simulink model "vrguiJP_R2012b_wersja2"  (R2019b)
settings: Solver=FixedStepDiscrete  StartTime=0.0  StopTime=inf  RelTol=1e-3  EnableMultiTasking=on
undefined symbols (not defined in the file): gray, pause, strel
libraries: visionanalysis x3, visiontextngfix x2, visionstatistics x1, visionmorphops x1, dspvision x1, visiongeotforms x1
settings Model: Creator=Tomek  LastModifiedBy=fw2ty
settings DataIOCC: LimitDataPoints=on  SaveFormat=Array  SignalLoggingSaveFormat=ModelDataLogs  ReturnWorkspaceOutputs=off
settings OptimizationCC: ExpressionDepthLimit=2147483647  InitFltsAndDblsToZero=on  LifeSpan=inf
settings DebuggingCC: SaveWithParameterizedLinksMsg=none  UnderspecifiedInitializationDetection=Classic  MergeDetectMultiDrivingBlocksExec=none  SignalResolutionControl=TryResolveAllWithWarning  MultiTaskDSMMsg=warning  MultiTaskCondExecSysMsg=none  FcnCallInpInsideContextMsg=warning  StateNameClashWarn=warning  SFUnexpectedBacktrackingDiag=warning  SFNoUnconditionalDefaultTransitionDiag=warning  SFExecutionAtInitializationDiag=none  ArithmeticOperatorsInVariantConditions=warning
settings HardwareCC: ProdBitPerPointer=32  ProdBitPerSizeT=32  ProdBitPerPtrDiffT=32  ProdLargestAtomicFloat=None  ProdIntDivRoundTo=Undefined  ProdEndianess=Unspecified  ProdWordSize=32  ProdHWDeviceType=32-bit Generic  TargetHWDeviceType=32-bit Generic  TargetUnknown=on  ProdEqTarget=off
settings ModelReferenceCC: PropagateSignalLabelsOutOfModel=off
settings SFSimCC: SimUseLocalCustomCode=off  SimParseCustomCode=off  CustomCodeUndefinedFunction=UseInterfaceOnly
settings RTWCC: RTWUseLocalCustomCode=off
settings CodeAppCC: StateflowObjectComments=on
settings GRTTargetCC: TargetFcnLib=ansi_tfl_tmw.mat  TargetLangStandard=C89/C90 (ANSI)  GeneratePreprocessorConditionals=Disable all  CombineOutputUpdateFcns=off  GRTInterface=on
settings ConfigComp: CovMetricSettings=dw  CovHtmlReporting=on  CovSaveCumulativeToWorkspaceVar=on  CovSaveSingleToWorkspaceVar=on  CovExternalEMLEnable=off

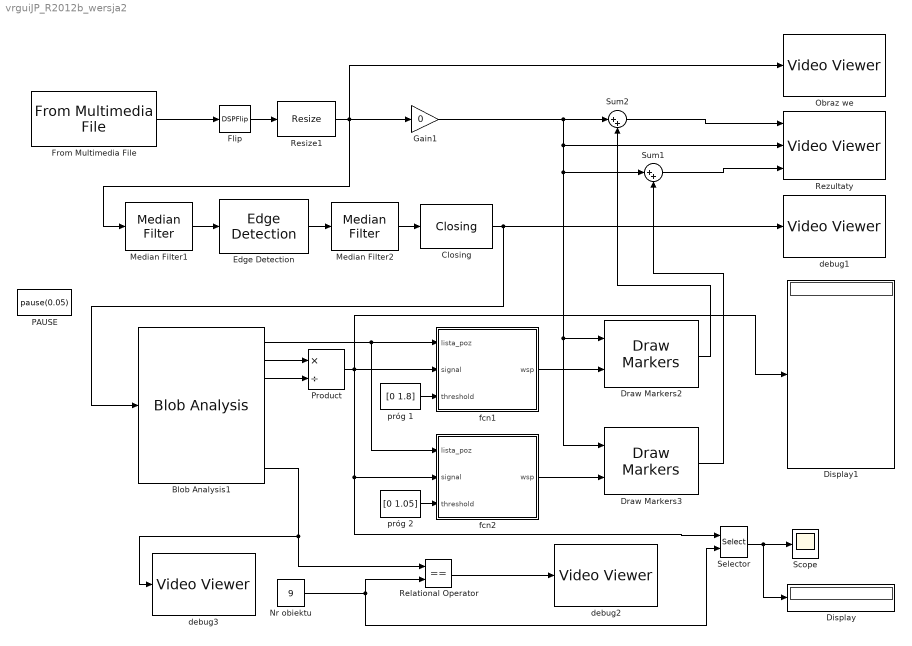
== system vrguiJP_R2012b_wersja2 ==
  Blob Analysis1 : visionstatistics/Blob Analysis  Tag=vipblks_row_conv  area=off  centroid=on  bBox=off  majorAxis=on  minorAxis=on  angle=off  eccentricity=on  equivDiameterSq=on  extent=on  perimeter=on  outDT=double  conn=8  isLabel=on  maxBlobs=10  warnIfNumBlobsExceeded=on  isCount=off  useMinArea=on  minArea=45  useMaxArea=off  maxArea=intmax('uint32')  excludeBorderBlob=on  isOutVarDim=off  isFill=on  fillValues=-1  roundingMode=Floor  overflowMode=off  prodOutputMode=Binary point scaling  prodOutputWordLength=32  prodOutputFracLength=16  prodOutputSlope=2^-16  accumMode=Binary point scaling  accumWordLength=32  accumFracLength=0  accumSlope=2^0  outputMode=Binary point scaling  outputWordLength=32  outputFracLength=16  outputSlope=2^-16  memorySlope=2^-16  firstCoeffMode=Binary point scaling  firstCoeffWordLength=16  firstCoeffFracLength=14  firstCoeffSlope=2^-14  secondCoeffMode=Binary point scaling  secondCoeffWordLength=32  secondCoeffFracLength=16  secondCoeffSlope=2^-16
      settings: SourceProductName=Computer Vision Toolbox
  Closing : visionmorphops/Closing  nhoodsrc=Specify via dialog  strel=strel('line',5,45)
      settings: SourceProductName=Computer Vision Toolbox  SourceProductBaseCode=VP
  Display : Display
  Display1 : Display
  Draw Markers2 : visiontextngfix/Draw Markers  shape=Circle  size=10  fill=on  fillClrSource=Specify via dialog  display=White  intensity=200  color=[200 255 100]  opacity=0.5  viewport=Entire image  antialiasing=off  inType=Obsolete  imagePorts=One multidimensional signal  roundingMode=Floor  overflowMode=off  memoryMode=Specify word length  memoryWordLength=16  memoryFracLength=14  memorySlope=2^-14  prodOutputMode=Binary point scaling  prodOutputWordLength=32  prodOutputFracLength=14  prodOutputSlope=2^-14  accumSlope=2^-14
      settings: SourceProductName=Computer Vision Toolbox  SourceProductBaseCode=VP
  Draw Markers3 : visiontextngfix/Draw Markers  shape=Circle  size=10  fill=on  fillClrSource=Specify via dialog  display=White  intensity=200  color=[200 255 100]  opacity=0.5  viewport=Entire image  antialiasing=off  inType=Obsolete  imagePorts=One multidimensional signal  roundingMode=Floor  overflowMode=off  memoryMode=Specify word length  memoryWordLength=16  memoryFracLength=14  memorySlope=2^-14  prodOutputMode=Binary point scaling  prodOutputWordLength=32  prodOutputFracLength=14  prodOutputSlope=2^-14  accumSlope=2^-14
      settings: SourceProductName=Computer Vision Toolbox  SourceProductBaseCode=VP
  Edge Detection : visionanalysis/Edge Detection  method=Sobel  outputType=Binary image  userDefinedThreshold=off  thresholdSource=Input port  threshold=20  thresholdTuning=12  edgeThinning=off  threshold_canny=[0.25 0.60]  autoPercent=70  sigma=1  roundingMode=Floor  overflowMode=off  prodOutputMode=Binary point scaling  prodOutputWordLength=32  prodOutputFracLength=8  prodOutputSlope=2^-8  accumSlope=2^-8  outputSlope=2^-4
      settings: SourceProductName=Computer Vision Toolbox  SourceProductBaseCode=VP
  Flip : DSPFlip
  From Multimedia File : dspvision/From Multimedia File  inputFilename=video1.avi  readRange=[1 Inf]  loop=on  numPlays=inf  outputStreams=Video only  videoDataType=single  audioDataType=int16  inheritSampleTime=off  userDefinedSampleTime=1  noAudioOutput=off  isIntensityVideo=off  fourcc=Intensity  colorVideoFormat=One multidimensional signal  outputEOF=off  dataOrg=Column-major  audioFrameSize=1024  computeAudioFrameSize=off  outSamplingMode=Sample based
      settings: SourceProductName=DSP System Toolbox  SourceProductBaseCode=DS
  Gain1 : Gain  Gain=0
  Median Filter1 : visionanalysis/Median Filter  nghbood=[3 3]  outSize=Same as input port I  padType=Constant  padSrc=Specify via dialog  padVal=0  roundingMode=Floor  overflowMode=off  prodOutputSlope=2^-30  accumSlope=2^-30  outputSlope=2^-15
      settings: SourceProductName=Computer Vision Toolbox  SourceProductBaseCode=VP
  Median Filter2 : visionanalysis/Median Filter  nghbood=[3 3]  outSize=Same as input port I  padType=Constant  padSrc=Specify via dialog  padVal=0  roundingMode=Floor  overflowMode=off  prodOutputSlope=2^-30  accumSlope=2^-30  outputSlope=2^-15
      settings: SourceProductName=Computer Vision Toolbox  SourceProductBaseCode=VP
  Nr obiektu : Constant  Value=9
  Obraz we : VideoViewer  colormapValue=gray(256)  FigPos=[1062 567 260 221]
  PAUSE : MATLABFcn  MATLABFcn=pause(0.05)  OutputDimensions=0
  Product : Product  Inputs=*/  RndMeth=Zero
  Relational Operator : RelationalOperator  Operator===  OutDataTypeStr=boolean  RndMeth=Nearest
  Resize1 : visiongeotforms/Resize  specify=Output size as a percentage of input size  rfactor=[100 100]  outCols=25  outRows=25  outRowsCols=[25 35]  interp_method=Bilinear  antialias=on  useROI=off  roiFlag=off  roundingMode=Nearest  overflowMode=on  prodOutputMode=Binary point scaling  prodOutputWordLength=32  prodOutputFracLength=10  prodOutputSlope=2^-10  accumSlope=2^-10  outputSlope=2^-10
      settings: SourceProductName=Computer Vision Toolbox  SourceProductBaseCode=VP
  Rezultaty : VideoViewer  imagePorts=separate color signals  colormapValue=gray(256)  FigPos=[1126 823 260 220]
  Scope : Scope
  Selector : Selector  IndexOptions=Index vector (port)  Indices=1  OutputSizes=1
  Sum1 : Sum  Inputs=|++
  Sum2 : Sum  Inputs=|++
  debug1 : VideoViewer  colormapValue=gray(256)  FigPos=[657 821 270 222]
  debug2 : VideoViewer  colormapValue=gray(256)  FigPos=[1343 898 248 218]
  debug3 : VideoViewer  useColorMap=on  specRange=on  maxInputVal=10  FigPos=[1616 900 262 220]
  fcn1 : MATLAB Function  TreatAsAtomicUnit=on
  fcn2 : MATLAB Function  TreatAsAtomicUnit=on
  próg 1 : Constant  Value=[0 1.8]
  próg 2 : Constant  Value=[0 1.05]
  wires:
  From Multimedia File/1 -> Flip/1
  Flip/1 -> Resize1/1
  Product/1 -> fcn2/2(signal), Selector/1, Display1/1, fcn1/2(signal)
  Blob Analysis1/1 -> fcn2/1(lista_poz), fcn1/1(lista_poz)
  Blob Analysis1/2 -> Product/1
  Blob Analysis1/3 -> Product/2
  Resize1/1 -> Obraz we/1, Gain1/1, Median Filter1/1
  Median Filter2/1 -> Closing/1
  Edge Detection/1 -> Median Filter2/1
  Median Filter1/1 -> Edge Detection/1
  fcn2/1(wsp) -> Draw Markers3/2
  Closing/1 -> Blob Analysis1/1, debug1/1
  Gain1/1 -> Sum2/1, Draw Markers3/1, Draw Markers2/1, Sum1/1, Rezultaty/2
  fcn1/1(wsp) -> Draw Markers2/2
  Sum1/1 -> Rezultaty/3
  Sum2/1 -> Rezultaty/1
  Draw Markers2/1 -> Sum2/2
  Draw Markers3/1 -> Sum1/2
  Selector/1 -> Display/1, Scope/1
  Relational Operator/1 -> debug2/1
  Blob Analysis1/8 -> debug3/1, Relational Operator/1
  Nr obiektu/1 -> Selector/2, Relational Operator/2
  próg 1/1 -> fcn1/3(threshold)
  próg 2/1 -> fcn2/3(threshold)

== matlab function vrguiJP_R2012b_wersja2/fcn2 ==
  data: lista_poz input; signal input; wsp output; threshold input
function wsp = fcn(lista_poz, signal, threshold)
%--------------------------------------------------------------------------
% Nazwa funkcji: fnc
% 
% Przeznaczenie:
%   Funkcja porownuje sygnał "signal" z zadanym progiem.
% 
% Argumenty funkcji:
%   (I) lista_poz - macierz zawierajaca pozycje srodkow ciezkosci elementow
%   (I) signal      - sygnał do porównania
%   (I) threshold   - próg, dwuelementowy wektor <min,max)
%
% Funkcja zwraca:
%   (O) wsp       - macierz zawierajaca pozycje srodka ciezkosci obiektu 
%                   jezeli element spelnia zadany warunek, badz wspolrzedne 
%                   (-100, -100) w przeciwnym wypadku
% Autor:
%   Jaromir Przybylo, R2012b
%
% Data napisania funkcji:
%   27.09.2018
%--------------------------------------------------------------------------

n1=size(lista_poz,1);
A=-100*ones(n1,2);

for R = 1:n1  
    if (signal(R) >= threshold(1)) & (signal(R) < threshold(2))
        A(R,:) = lista_poz(R,:);
    end
end

wsp = int16(A);

== matlab function vrguiJP_R2012b_wersja2/fcn1 ==
  data: lista_poz input; signal input; wsp output; threshold input
function wsp = fcn(lista_poz, signal, threshold)
%--------------------------------------------------------------------------
% Nazwa funkcji: fnc
% 
% Przeznaczenie:
%   Funkcja porownuje sygnał "signal" z zadanym progiem.
% 
% Argumenty funkcji:
%   (I) lista_poz - macierz zawierajaca pozycje srodkow ciezkosci elementow
%   (I) signal      - sygnał do porównania
%   (I) threshold   - próg, dwuelementowy wektor <min,max)
%
% Funkcja zwraca:
%   (O) wsp       - macierz zawierajaca pozycje srodka ciezkosci obiektu 
%                   jezeli element spelnia zadany warunek, badz wspolrzedne 
%                   (-100, -100) w przeciwnym wypadku
% Autor:
%   Jaromir Przybylo, R2012b
%
% Data napisania funkcji:
%   27.09.2018
%--------------------------------------------------------------------------

n1=size(lista_poz,1);
A=-100*ones(n1,2);

for R = 1:n1  
    if (signal(R) >= threshold(1)) & (signal(R) < threshold(2))
        A(R,:) = lista_poz(R,:);
    end
end

wsp = int16(A);
